simulink model "mainprueba3"  (R2016b)
settings: Solver=VariableStepAuto  StartTime=0.0  StopTime=10.0  MaxStep=0.2  RelTol=1e-2
undefined symbols (not defined in the file): checks, Earth, initialValues, LD, Newton, Raphson, WGS84
libraries: aerolibasang x5, aerolibutil x5, simulink x5, aerolibbdyn x3, aerolibatmos2 x1, aerolibobsolete x1, aerolibadyn x1, aerolibadynsys x1, aerolib6dof2 x1, aerolibtransform2 x1
(part 1 of 2)
settings Model: Creator=Uxío  LastModifiedBy=Uxío
settings DebuggingCC: ReadBeforeWriteMsg=DisableAll  WriteAfterWriteMsg=DisableAll  WriteAfterReadMsg=DisableAll  MultiTaskDSMMsg=none

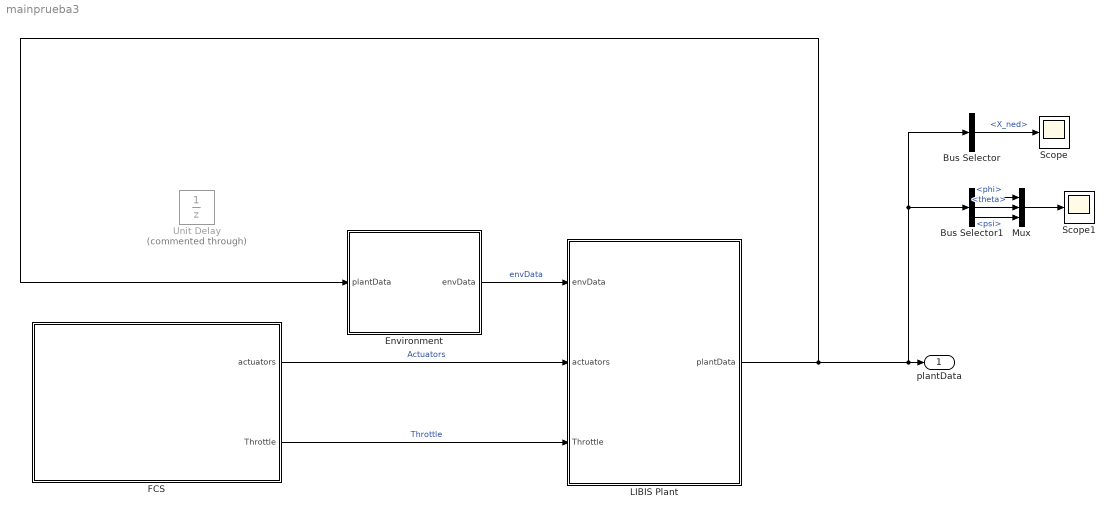
== system mainprueba3 ==
  Bus Selector : BusSelector  OutputSignals=X_ned
  Bus Selector1 : BusSelector  OutputSignals=Euler.phi,Euler.theta,Euler.psi
  Environment : Subsystem
      mask Display:
      | imageName='Wind.png';
      | currentPath=get_param(bdroot, 'FileName');
      | positions=strfind(currentPath,'\');
      | imagePath=strcat(currentPath(1:positions(end-1)),'graphics\',imageName);
      | image(imagePath);
  FCS : Subsystem
      mask Display:
      | imageName='FCS.png';
      | currentPath=get_param(bdroot, 'FileName');
      | positions=strfind(currentPath,'\');
      | imagePath=strcat(currentPath(1:positions(end-1)),'graphics\',imageName);
      | image(imagePath);
  LIBIS Plant : Subsystem
      mask Display:
      | imageName='LIBIS_Plant.jpg';
      | currentPath=get_param(bdroot, 'FileName');
      | positions=strfind(currentPath,'\');
      | imagePath=strcat(currentPath(1:positions(end-1)),'graphics\',imageName);
      | image(imagePath);
  Mux : Mux  Inputs=3
  Scope : Scope
  Scope1 : Scope
  Unit Delay : UnitDelay  Commented=through  SampleTime=-1
  plantData : Outport
  wires:
  LIBIS Plant/1(plantData) -> Environment/1(plantData), Bus Selector1/1, Bus Selector/1, plantData/1
  Environment/1(envData) -> LIBIS Plant/1(envData)  "envData"
  FCS/1(actuators) -> LIBIS Plant/2(actuators)  "Actuators"
  FCS/2(Throttle) -> LIBIS Plant/3(Throttle)  "Throttle"
  Bus Selector/1 -> Scope/1  "<X_ned>"
  Bus Selector1/1 -> Mux/1  "<phi>"
  Bus Selector1/2 -> Mux/2  "<theta>"
  Bus Selector1/3 -> Mux/3  "<psi>"
  Mux/1 -> Scope1/1

== system mainprueba3/Environment ==
  plantData : Inport
  Bus Selector : BusSelector  OutputSignals=X_ned,LLA.Altitude_m,V_ned,DCM_body_earth,LLA.Latitude_deg
  COESA Atmosphere Model : aerolibatmos2/COESA Atmosphere Model  units=Metric (MKS)  spec=1976 COESA-extended U.S. Standard Atmosphere  model=Profile  profile_var=High temperature  profile_percent=1%  profile_alt=5 km (16404 ft)  envelope_var=High temperature  envelope_percent=1%  action=Warning
  Gravity in Earth Axes : Gain  Gain=[0 0 LD.Inertia.mass]  SaturateOnIntegerOverflow=on  OutDataTypeStr=Inherit: Same as input  ParamDataTypeStr=Inherit: Same as input
  Math Function : Math  Operator=transpose  SaturateOnIntegerOverflow=on
  Terrain : Subsystem
  To Body Axes : Product  Multiplication=Matrix(*)  SaturateOnIntegerOverflow=on  InputSameDT=on  OutDataTypeStr=Inherit: Same as first input
  WGS84 Gravity Model : aerolibobsolete/WGS84 Gravity Model  model=WGS84 Taylor Series  units=Metric (MKS)  no_atmos=on  precessing=on  month=February  day=1  year=2000  no_centrifugal=on  action=Warning
  Wind Models : Subsystem
  envDataBus : BusCreator  Inputs='h_ground','windVelocity','windOmega','T','a','P','AirDensity','Fg'  OutDataTypeStr=Bus: envDataBus  NonVirtualBus=on
  envData : Outport  InitialOutput=0
  wires:
  [Altitude] -> COESA Atmosphere Model/1
  Bus Selector/4 -> Wind Models/3(DCM_be), To Body Axes/1  "<DCM_body_earth>"
  Bus Selector/5 -> WGS84 Gravity Model/2  "<Latitude_deg>"
  Bus Selector/3 -> Wind Models/1(Ve)  "<V_ned>"
  [Altitude] -> WGS84 Gravity Model/1
  envDataBus/1 -> envData/1  "envData"
  To Body Axes/1 -> envDataBus/8  "Fg"
  Wind Models/2(windOmega) -> envDataBus/3  "windOmega"
  Bus Selector/1 -> Terrain/1(Xe)  "<X_ned>"
  WGS84 Gravity Model/1 -> Gravity in Earth Axes/1
  COESA Atmosphere Model/3 -> envDataBus/6  "P"
  COESA Atmosphere Model/2 -> envDataBus/5  "a"
  Wind Models/1(windVelocity) -> envDataBus/2  "windVelocity"
  [Altitude] -> Wind Models/2(Altitude)
  COESA Atmosphere Model/1 -> envDataBus/4  "T"
  COESA Atmosphere Model/4 -> envDataBus/7  "AirDensity"
  plantData/1 -> Bus Selector/1
  Terrain/1(hground) -> envDataBus/1  "h_ground"
  Bus Selector/2 -> [Altitude]  "<Altitude_m>"
  Gravity in Earth Axes/1 -> Math Function/1
  Math Function/1 -> To Body Axes/2

== system mainprueba3/FCS ==
  Bus Creator : BusCreator  Inputs=4
  Bus Creator1 : BusCreator  Inputs=5
  Constant{,1..4} (5 alike) : Constant  Value=0
  Constant{5..8} (4 alike) : Constant
  actuators : Outport
  Throttle : Outport  Port=2
  wires:
  Bus Creator/1 -> actuators/1  "actuators"
  Constant/1 -> Bus Creator/1  "deltae"
  Constant1/1 -> Bus Creator/2  "deltar"
  Constant2/1 -> Bus Creator/3  "deltafr"
  Constant3/1 -> Bus Creator/4  "deltafl"
  Constant4/1 -> Bus Creator1/1  "Throttle1"
  Constant5/1 -> Bus Creator1/2  "Throttle2"
  Constant6/1 -> Bus Creator1/3  "Throttle3"
  Constant7/1 -> Bus Creator1/4  "Throttle4"
  Constant8/1 -> Bus Creator1/5  "Throttle5"
  Bus Creator1/1 -> Throttle/1

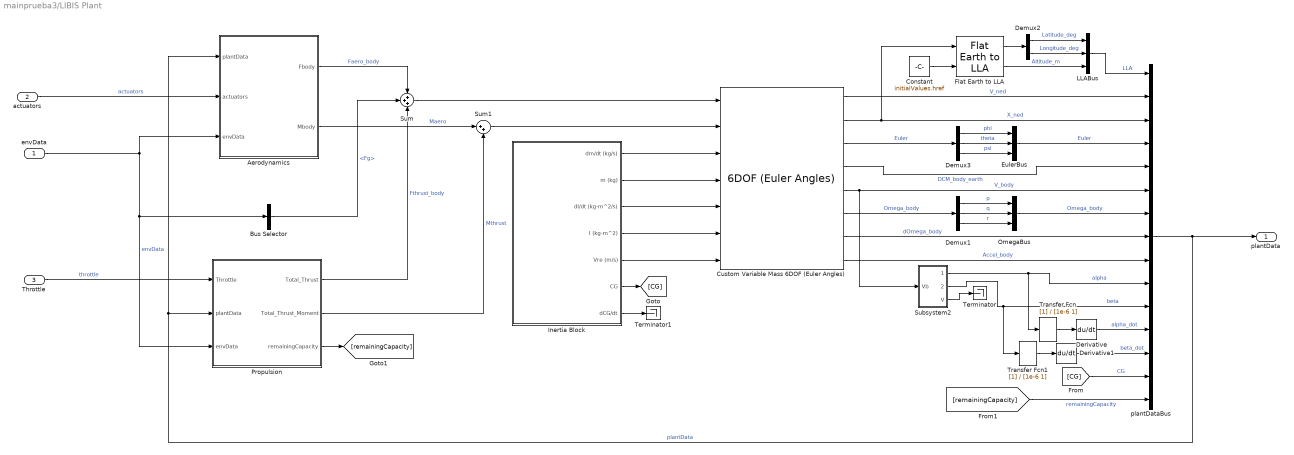
== system mainprueba3/LIBIS Plant ==
  envData : Inport
  actuators : Inport  Port=2
  Throttle : Inport  Port=3
  Aerodynamics : Subsystem
  Bus Selector : BusSelector  OutputSignals=Fg
  Constant : Constant  Value=initialValues.href
  Custom Variable Mass 6DOF (Euler Angles) : aerolib6dof2/6DOF (Euler Angles)  units=Metric (MKS)  mtype=Custom Variable  rep=Euler Angles  xme_0=[initialValues.Xe0 initialValues.Ye0 initialValues.Ze0]  Vm_0=[initialValues.u0 initialValues.v0 initialValues.w0]  eul_0=[initialValues.roll0 initialValues.pitch0 initialValues.yaw0]  pm_0=[initialValues.p0 initialValues.q0 initialValues.r0]  mass_0=1.0  mass_e=0.5  mass_f=2.0  inertia=eye(3)  inertia_e=eye(3)  inertia_f=2*eye(3)  k_quat=1.0  vre_flag=on
  Demux1 : Demux  Outputs=3
  Demux2 : Demux  Outputs=2
  Demux3 : Demux  Outputs=3
  Derivative : Derivative
  Derivative1 : Derivative
  EulerBus : BusCreator  Inputs='phi','theta','psi'  OutDataTypeStr=Bus: EulerBus  NonVirtualBus=on
  Flat Earth to LLA : aerolibtransform2/Flat Earth to LLA  units=Metric (MKS)  ptype=Earth (WGS84)  F=1/298.257223563  R=6378137  LL0=initialValues.LatLong0  psi=initialValues.heading0
  Inertia Block : Subsystem
      mask Display:
      | imageName='Moment_of_inertia.png';
      | currentPath=get_param(bdroot, 'FileName');
      | positions=strfind(currentPath,'\');
      | imagePath=strcat(currentPath(1:positions(end-1)),'graphics\',imageName);
      | image(imagePath);
  LLABus : BusCreator  Inputs='Latitude_deg','Longitude_deg','Altitude_m'  OutDataTypeStr=Bus: LLABus  NonVirtualBus=on
  OmegaBus : BusCreator  Inputs='p','q','r'  OutDataTypeStr=Bus: OmegaBus  NonVirtualBus=on
  Propulsion : Subsystem
  Subsystem2 : Subsystem
  Sum : Sum  Inputs=+++
  Sum1 : Sum  Inputs=|++
  Terminator : Terminator
  Terminator1 : Terminator
  Transfer Fcn : TransferFcn  Denominator=[1e-6 1]
  Transfer Fcn1 : TransferFcn  Denominator=[1e-6 1]
  plantDataBus : BusCreator  Inputs='LLA','V_ned','X_ned','Euler','DCM_body_earth','V_body','Omega_body','dOmega_body','Accel_body','alpha','beta','alpha_dot','beta_dot','CG','remainingCapacity'  OutDataTypeStr=Bus: plantDataBus  NonVirtualBus=on
  plantData : Outport
  wires:
  envData/1 -> Aerodynamics/3(envData), Propulsion/3(envData), Bus Selector/1  "envData"
  Inertia Block/4(I (kg-m^2)) -> Custom Variable Mass 6DOF (Euler Angles)/6
  Derivative1/1 -> plantDataBus/13  "beta_dot"
  plantDataBus/1 -> plantData/1, Propulsion/2(plantData), Aerodynamics/1(plantData)  "plantData"
  Flat Earth to LLA/2 -> LLABus/3  "Altitude_m"
  Custom Variable Mass 6DOF (Euler Angles)/2 -> plantDataBus/3, Flat Earth to LLA/1  "X_ned"
  Subsystem2/3(V) -> Terminator/1
  Custom Variable Mass 6DOF (Euler Angles)/3 -> Demux3/1  "Euler"
  EulerBus/1 -> plantDataBus/4  "Euler"
  Flat Earth to LLA/1 -> Demux2/1
  Demux2/1 -> LLABus/1  "Latitude_deg"
  Inertia Block/2(m (kg)) -> Custom Variable Mass 6DOF (Euler Angles)/4
  Inertia Block/5(Vre (m/s)) -> Custom Variable Mass 6DOF (Euler Angles)/7
  Custom Variable Mass 6DOF (Euler Angles)/5 -> Subsystem2/1(Vb), plantDataBus/6  "V_body"
  Inertia Block/7(dCG/dt) -> Terminator1/1
  [CG] -> plantDataBus/14  "CG"
  Custom Variable Mass 6DOF (Euler Angles)/4 -> plantDataBus/5  "DCM_body_earth"
  Inertia Block/3(dI/dt (kg-m^2/s)) -> Custom Variable Mass 6DOF (Euler Angles)/5
  LLABus/1 -> plantDataBus/1  "LLA"
  Custom Variable Mass 6DOF (Euler Angles)/8 -> plantDataBus/9  "Accel_body"
  Subsystem2/1(Alpha) -> Transfer Fcn/1, plantDataBus/10  "alpha"
  Demux3/1 -> EulerBus/1  "phi"
  Demux3/3 -> EulerBus/3  "psi"
  Inertia Block/6(CG) -> [CG]
  Inertia Block/1(dm/dt (kg/s)) -> Custom Variable Mass 6DOF (Euler Angles)/3
  Constant/1 -> Flat Earth to LLA/2
  Demux2/2 -> LLABus/2  "Longitude_deg"
  Custom Variable Mass 6DOF (Euler Angles)/7 -> plantDataBus/8  "dOmega_body"
  Subsystem2/2(Beta) -> Transfer Fcn1/1, plantDataBus/11  "beta"
  Demux3/2 -> EulerBus/2  "theta"
  Derivative/1 -> plantDataBus/12  "alpha_dot"
  Custom Variable Mass 6DOF (Euler Angles)/1 -> plantDataBus/2  "V_ned"
  OmegaBus/1 -> plantDataBus/7  "Omega_body"
  Custom Variable Mass 6DOF (Euler Angles)/6 -> Demux1/1  "Omega_body"
  Demux1/2 -> OmegaBus/2  "q"
  Demux1/1 -> OmegaBus/1  "p"
  Demux1/3 -> OmegaBus/3  "r"
  Aerodynamics/1(Fbody) -> Sum/1  "Faero_body"
  Sum1/1 -> Custom Variable Mass 6DOF (Euler Angles)/2
  Aerodynamics/2(Mbody) -> Sum1/1  "Maero"
  Propulsion/2(Total_Thrust_Moment) -> Sum1/2  "Mthrust"
  actuators/1 -> Aerodynamics/2(actuators)  "actuators"
  Throttle/1 -> Propulsion/1(Throttle)  "throttle"
  Propulsion/3(remainingCapacity) -> [remainingCapacity]
  [remainingCapacity] -> plantDataBus/15  "remainingCapacity"
  Propulsion/1(Total_Thrust) -> Sum/3  "Fthrust_body"
  Bus Selector/1 -> Sum/2  "<Fg>"
  Sum/1 -> Custom Variable Mass 6DOF (Euler Angles)/1
  Transfer Fcn1/1 -> Derivative1/1
  Transfer Fcn/1 -> Derivative/1

== system mainprueba3/Environment/Terrain ==
  note: This part of the system defines the interface for the terrain model that will be developed in detail later on.
  Xe : Inport
  Terminator : Terminator
  hground_value : Constant  Value=initialValues.href  OutDataTypeStr=double
  hground : Outport  Unit=m
  wires:
  Xe/1 -> Terminator/1
  hground_value/1 -> hground/1  "hground"

== system mainprueba3/Environment/Wind Models ==
  Ve : Inport
  Altitude : Inport  Port=2
  DCM_be : Inport  Port=3
  Constant : Constant  Value=[0,0,0]
  Constant1 : Constant  Value=[0,0,0]
  Dot Product : DotProduct  OutDataTypeStr=Inherit: Inherit via internal rule
  vt : Sqrt  SaturateOnIntegerOverflow=on
  windVelocity : Outport  Unit=m/s
  windOmega : Outport  Port=2  Unit=rad/second
  wires:
  DCM_be/1 -> [DCM]
  Altitude/1 -> [Altitude]
  vt/1 -> [Airspeed]  "Airspeed"
  Dot Product/1 -> vt/1
  Ve/1 -> Dot Product/2, Dot Product/1
  Constant/1 -> windVelocity/1
  Constant1/1 -> windOmega/1

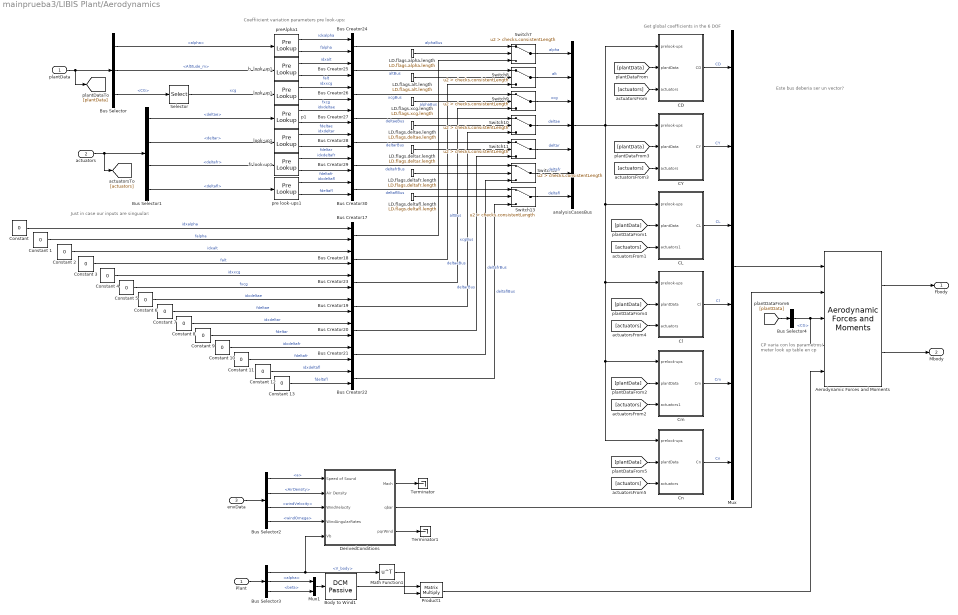
== system mainprueba3/LIBIS Plant/Aerodynamics ==
  note: Este bus deberia ser un vector?
  note: CP varia con los parametros! meter look up table en cp
  note: Just in case our inputs are singuular:
  note: Get global coefficients in the 6 DOF
  note: Coeffiicient variation parameters pre look-ups:
  plantData : Inport
  actuators : Inport  Port=2
  envData : Inport  Port=3
  " look-up1" : PreLookup  BreakpointsData=LD.xcg  BeginIndexSearchUsingPreviousIndexResult=on  IndexDataTypeStr=int32  FractionDataTypeStr=double
  "Aerodynamic Forces and Moments " : aerolibadyn/Aerodynamic Forces and Moments   inputAxes=Stability  outputForceAxes=Body  outputMomentAxes=Body  S=LD.sref  b=LD.blref  cbar=LD.cbar
  Body to Wind1 : aerolibadynsys/DCM Passive  SystemSampleTime=-1
  Bus Creator17 : BusCreator  Inputs='idxalpha','falpha'  OutDataTypeStr=Bus: alphaBus  NonVirtualBus=on
  Bus Creator18 : BusCreator  Inputs='idxalt','falt'  OutDataTypeStr=Bus: altBus  NonVirtualBus=on
  Bus Creator19 : BusCreator  Inputs='idxdeltae','fdeltae'  OutDataTypeStr=Bus: deltaeBus  NonVirtualBus=on
  Bus Creator20 : BusCreator  Inputs='idxdeltar','fdeltar'  OutDataTypeStr=Bus: deltarBus  NonVirtualBus=on
  Bus Creator21 : BusCreator  Inputs='idxdeltafr','fdeltafr'  OutDataTypeStr=Bus: deltafrBus  NonVirtualBus=on
  Bus Creator22 : BusCreator  Inputs='idxdeltafl','fdeltafl'  OutDataTypeStr=Bus: deltaflBus  NonVirtualBus=on
  Bus Creator23 : BusCreator  Inputs='idxxcg','fxcg'  OutDataTypeStr=Bus: xcgBus  NonVirtualBus=on
  Bus Creator24 : BusCreator  Inputs='idxalpha','falpha'  OutDataTypeStr=Bus: alphaBus  NonVirtualBus=on
  Bus Creator25 : BusCreator  Inputs='idxalt','falt'  OutDataTypeStr=Bus: altBus  NonVirtualBus=on
  Bus Creator26 : BusCreator  Inputs='idxxcg','fxcg'  OutDataTypeStr=Bus: xcgBus  NonVirtualBus=on
  Bus Creator27 : BusCreator  Inputs='idxdeltae','fdeltae'  OutDataTypeStr=Bus: deltaeBus  NonVirtualBus=on
  Bus Creator28 : BusCreator  Inputs='idxdeltar','fdeltar'  OutDataTypeStr=Bus: deltarBus  NonVirtualBus=on
  Bus Creator29 : BusCreator  Inputs='idxdeltafr','fdeltafr'  OutDataTypeStr=Bus: deltafrBus  NonVirtualBus=on
  Bus Creator30 : BusCreator  Inputs='idxdeltafl','fdeltafl'  OutDataTypeStr=Bus: deltaflBus  NonVirtualBus=on
  Bus Selector : BusSelector  OutputSignals=alpha,LLA.Altitude_m,CG
  Bus Selector1 : BusSelector  OutputSignals=deltae,deltar,deltafr,deltafl
  Bus Selector2 : BusSelector  OutputSignals=a,AirDensity,windVelocity,windOmega
  Bus Selector3 : BusSelector  OutputSignals=V_body,alpha,beta
  Bus Selector4 : BusSelector  OutputSignals=CG
  CD : Subsystem
  CL : Subsystem
  CY : Subsystem
  Cl : Subsystem
  Cm : Subsystem
  Cn : Subsystem
  Constant {,2,4,6,8,10,12} (7 alike) : Constant  Value=0  OutDataTypeStr=int32
  Constant {1,3,5,7,9,11,13} (7 alike) : Constant  Value=0
  DerivedConditions : Subsystem
  LD.flags.alpha.length : Constant  Value=LD.flags.alpha.length
  LD.flags.alt.length : Constant  Value=LD.flags.alt.length
  LD.flags.deltae.length : Constant  Value=LD.flags.deltae.length
  LD.flags.deltafl.length : Constant  Value=LD.flags.deltafl.length
  LD.flags.deltafr.length : Constant  Value=LD.flags.deltafr.length
  LD.flags.deltar.length : Constant  Value=LD.flags.deltar.length
  LD.flags.xcg.length : Constant  Value=LD.flags.xcg.length
  Math Function1 : Math  Operator=transpose  SaturateOnIntegerOverflow=on
  Mux : Mux  Inputs=6
  Mux1 : Mux  Inputs=2
  "Plant " : InportShadow
  Product1 : Product  Multiplication=Matrix(*)  RndMeth=Zero
  Selector : Selector  InputPortWidth=3  IndexOptions=Index vector (dialog)  Indices=[1 ]  OutputSizes=1
  Switch{7..13} (7 alike) : Switch  Criteria=u2 > Threshold  Threshold=checks.consistentLength
  Terminator : Terminator
  Terminator1 : Terminator
  analysisCasesBus : BusCreator  Inputs='alpha','alt','xcg','deltae','deltar','deltafr','deltafl'  OutDataTypeStr=Bus: analysisCasesBus  NonVirtualBus=on
  fr look-up1 : PreLookup  BreakpointsData=LD.deltafr  BeginIndexSearchUsingPreviousIndexResult=on  IndexDataTypeStr=int32  FractionDataTypeStr=double
  h  look-up1 : PreLookup  BreakpointsData=LD.alt  BeginIndexSearchUsingPreviousIndexResult=on  IndexDataTypeStr=int32  FractionDataTypeStr=double
  look-up1 : PreLookup  BreakpointsData=LD.deltar  BeginIndexSearchUsingPreviousIndexResult=on  IndexDataTypeStr=int32  FractionDataTypeStr=double
  p1 : PreLookup  BreakpointsData=LD.deltae  BeginIndexSearchUsingPreviousIndexResult=on  IndexDataTypeStr=int32  FractionDataTypeStr=double
  pre look-ups1 : PreLookup  BreakpointsData=LD.deltafl  BeginIndexSearchUsingPreviousIndexResult=on  IndexDataTypeStr=int32  FractionDataTypeStr=double
  preAlpha1 : PreLookup  BreakpointsData=LD.alpha  BeginIndexSearchUsingPreviousIndexResult=on  IndexDataTypeStr=int32  FractionDataTypeStr=double
  Fbody : Outport  Unit=N
  Mbody : Outport  Port=2  Unit=N*m
  wires:
  plantData/1 -> [plantData], Bus Selector/1
  Mux1/1 -> Body to Wind1/1
  preAlpha1/2 -> Bus Creator24/2  "falpha"
  preAlpha1/1 -> Bus Creator24/1  "idxalpha"
  h  look-up1/2 -> Bus Creator25/2  "falt"
  h  look-up1/1 -> Bus Creator25/1  "idxalt"
  " look-up1"/1 -> Bus Creator26/1  "idxxcg"
  " look-up1"/2 -> Bus Creator26/2  "fxcg"
  p1/2 -> Bus Creator27/2  "fdeltae"
  p1/1 -> Bus Creator27/1  "idxdeltae"
  look-up1/2 -> Bus Creator28/2  "fdeltar"
  look-up1/1 -> Bus Creator28/1  "idxdeltar"
  fr look-up1/2 -> Bus Creator29/2  "fdeltafr"
  fr look-up1/1 -> Bus Creator29/1  "idxdeltafr"
  pre look-ups1/1 -> Bus Creator30/1  "idxdeltafl"
  pre look-ups1/2 -> Bus Creator30/2  "fdeltafl"
  LD.flags.alpha.length/1 -> Switch7/2
  Bus Creator24/1 -> Switch7/1  "alphaBus"
  LD.flags.alt.length/1 -> Switch8/2
  Bus Creator25/1 -> Switch8/1  "altBus"
  LD.flags.xcg.length/1 -> Switch9/2
  Bus Creator26/1 -> Switch9/1  "xcgBus"
  LD.flags.deltae.length/1 -> Switch10/2
  Bus Creator27/1 -> Switch10/1  "deltaeBus"
  LD.flags.deltar.length/1 -> Switch11/2
  Bus Creator28/1 -> Switch11/1  "deltarBus"
  LD.flags.deltafr.length/1 -> Switch12/2
  Bus Creator29/1 -> Switch12/1  "deltafrBus"
  LD.flags.deltafl.length/1 -> Switch13/2
  Bus Creator30/1 -> Switch13/1  "deltaflBus"
  Bus Creator17/1 -> Switch7/3  "alphaBus"
  Bus Creator18/1 -> Switch8/3  "altBus"
  Bus Creator23/1 -> Switch9/3  "xcgBus"
  Bus Creator19/1 -> Switch10/3  "deltaeBus"
  Bus Creator20/1 -> Switch11/3  "deltarBus"
  Bus Creator21/1 -> Switch12/3  "deltafrBus"
  Bus Creator22/1 -> Switch13/3  "deltaflBus"
  Switch7/1 -> analysisCasesBus/1  "alpha"
  Switch8/1 -> analysisCasesBus/2  "alt"
  Switch9/1 -> analysisCasesBus/3  "xcg"
  Switch10/1 -> analysisCasesBus/4  "deltae"
  Switch11/1 -> analysisCasesBus/5  "deltar"
  Switch12/1 -> analysisCasesBus/6  "deltafr"
  Switch13/1 -> analysisCasesBus/7  "deltafl"
  Constant 1/1 -> Bus Creator17/2  "falpha"
  "Constant "/1 -> Bus Creator17/1  "idxalpha"
  Constant 3/1 -> Bus Creator18/2  "falt"
  Constant 2/1 -> Bus Creator18/1  "idxalt"
  Constant 4/1 -> Bus Creator23/1  "idxxcg"
  Constant 5/1 -> Bus Creator23/2  "fxcg"
  Constant 7/1 -> Bus Creator19/2  "fdeltae"
  Constant 6/1 -> Bus Creator19/1  "idxdeltae"
  Constant 9/1 -> Bus Creator20/2  "fdeltar"
  Constant 8/1 -> Bus Creator20/1  "idxdeltar"
  Constant 11/1 -> Bus Creator21/2  "fdeltafr"
  Constant 10/1 -> Bus Creator21/1  "idxdeltafr"
  Constant 12/1 -> Bus Creator22/1  "idxdeltafl"
  Constant 13/1 -> Bus Creator22/2  "fdeltafl"
  analysisCasesBus/1 -> CD/1(prelook-ups), CY/1(prelook-ups), CL/1(prelook-ups), Cl/1(prelook-ups), Cm/1(prelook-ups), Cn/1(prelook-ups)
  Bus Selector/1 -> preAlpha1/1  "<alpha>"
  Bus Selector/2 -> h  look-up1/1  "<Altitude_m>"
  Bus Selector/3 -> Selector/1  "<CG>"
  Selector/1 -> " look-up1"/1  "xcg"
  actuators/1 -> [actuators], Bus Selector1/1
  Bus Selector1/1 -> p1/1  "<deltae>"
  Bus Selector1/2 -> look-up1/1  "<deltar>"
  Bus Selector1/3 -> fr look-up1/1  "<deltafr>"
  Bus Selector1/4 -> pre look-ups1/1  "<deltafl>"
  [plantData] -> CD/2(plantData)
  [actuators] -> CD/3(actuators)
  [plantData] -> CL/2(plantData)
  [plantData] -> Cm/2(plantData)
  [plantData] -> CY/2(plantData)
  [actuators] -> CY/3(actuators)
  [plantData] -> Cl/2(plantData)
  [actuators] -> Cl/3(actuators)
  [plantData] -> Cn/2(plantData)
  [actuators] -> Cn/3(actuators)
  Cn/1(Cn) -> Mux/6  "Cn"
  Cl/1(Cl) -> Mux/4  "Cl"
  CL/1(CL) -> Mux/3  "CL"
  CY/1(CY) -> Mux/2  "CY"
  CD/1(CD) -> Mux/1  "CD"
  Cm/1(Cm) -> Mux/5  "Cm"
  Mux/1 -> "Aerodynamic Forces and Moments "/1
  "Aerodynamic Forces and Moments "/1 -> Fbody/1
  "Aerodynamic Forces and Moments "/2 -> Mbody/1
  envData/1 -> Bus Selector2/1
  Bus Selector2/1 -> DerivedConditions/1(Speed of Sound)  "<a>"
  Bus Selector2/2 -> DerivedConditions/2(Air Density)  "<AirDensity>"
  Bus Selector2/3 -> DerivedConditions/3(WindVelocity)  "<windVelocity>"
  Bus Selector2/4 -> DerivedConditions/4(WindAngularRates)  "<windOmega>"
  "Plant "/1 -> Bus Selector3/1
  Bus Selector3/1 -> DerivedConditions/5(Vb), Math Function1/1  "<V_body>"
  DerivedConditions/1(Mach) -> Terminator/1
  DerivedConditions/3("pqrWind ") -> Terminator1/1
  DerivedConditions/2(qbar) -> "Aerodynamic Forces and Moments "/2
  Product1/1 -> "Aerodynamic Forces and Moments "/5
  Bus Selector3/2 -> Mux1/1  "<alpha>"
  Bus Selector3/3 -> Mux1/2  "<beta>"
  [plantData] -> Bus Selector4/1
  Bus Selector4/1 -> "Aerodynamic Forces and Moments "/4, "Aerodynamic Forces and Moments "/3  "<CG>"
  [actuators] -> CL/3(actuators1)
  [actuators] -> Cm/3(actuators1)
  Body to Wind1/1 -> Product1/1
  Math Function1/1 -> Product1/2

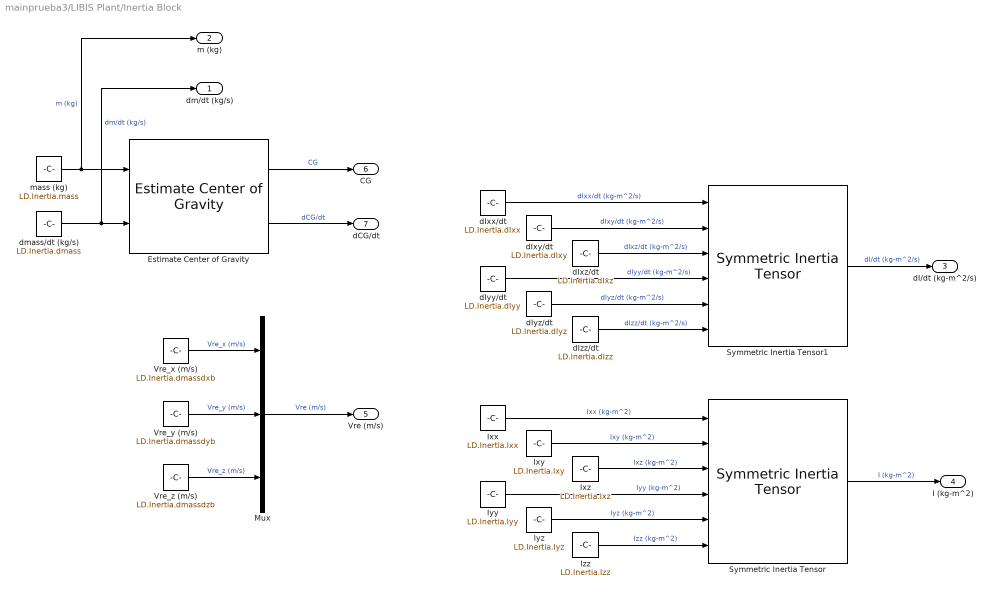
== system mainprueba3/LIBIS Plant/Inertia Block ==
  Estimate Center of Gravity : aerolibbdyn/Estimate Center of Gravity  fmass=LD.Inertia.fullMass  emass=LD.Inertia.emptyMass-1  fcg=LD.Inertia.fullCG  ecg=LD.Inertia.emptyCG
  Ixx : Constant  Value=LD.Inertia.Ixx
  Ixy : Constant  Value=LD.Inertia.Ixy
  Ixz : Constant  Value=LD.Inertia.Ixz
  Iyy : Constant  Value=LD.Inertia.Iyy
  Iyz : Constant  Value=LD.Inertia.Iyz
  Izz : Constant  Value=LD.Inertia.Izz
  Mux : Mux  Inputs=3
  Symmetric Inertia Tensor : aerolibbdyn/Symmetric Inertia Tensor
  Symmetric Inertia Tensor1 : aerolibbdyn/Symmetric Inertia Tensor
  Vre_x (m/s) : Constant  Value=LD.Inertia.dmassdxb
  Vre_y (m/s) : Constant  Value=LD.Inertia.dmassdyb
  Vre_z (m/s) : Constant  Value=LD.Inertia.dmassdzb
  dIxx/dt : Constant  Value=LD.Inertia.dIxx
  dIxy/dt : Constant  Value=LD.Inertia.dIxy
  dIxz/dt : Constant  Value=LD.Inertia.dIxz
  dIyy/dt : Constant  Value=LD.Inertia.dIyy
  dIyz/dt : Constant  Value=LD.Inertia.dIyz
  dIzz/dt : Constant  Value=LD.Inertia.dIzz
  dmass/dt (kg/s) : Constant  Value=LD.Inertia.dmass
  mass (kg) : Constant  Value=LD.Inertia.mass
  dm/dt (kg/s) : Outport  Unit=kg/s
  m (kg) : Outport  Port=2  Unit=kg
  dI/dt (kg-m^2/s) : Outport  Port=3  Unit=kg*meter^2/s
  I (kg-m^2) : Outport  Port=4  Unit=kg*meter*meter
  Vre (m/s) : Outport  Port=5  Unit=meter/s
  CG : Outport  Port=6
  dCG/dt : Outport  Port=7
  wires:
  Symmetric Inertia Tensor/1 -> I (kg-m^2)/1  "I (kg-m^2)"
  Symmetric Inertia Tensor1/1 -> dI/dt (kg-m^2/s)/1  "dI/dt (kg-m^2/s)"
  dIxx/dt/1 -> Symmetric Inertia Tensor1/1  "dIxx/dt (kg-m^2/s)"
  dIxz/dt/1 -> Symmetric Inertia Tensor1/3  "dIxz/dt (kg-m^2/s)"
  dIxy/dt/1 -> Symmetric Inertia Tensor1/2  "dIxy/dt (kg-m^2/s)"
  dIyy/dt/1 -> Symmetric Inertia Tensor1/4  "dIyy/dt (kg-m^2/s)"
  dIzz/dt/1 -> Symmetric Inertia Tensor1/6  "dIzz/dt (kg-m^2/s)"
  dIyz/dt/1 -> Symmetric Inertia Tensor1/5  "dIyz/dt (kg-m^2/s)"
  Ixx/1 -> Symmetric Inertia Tensor/1  "Ixx (kg-m^2)"
  Ixz/1 -> Symmetric Inertia Tensor/3  "Ixz (kg-m^2)"
  Ixy/1 -> Symmetric Inertia Tensor/2  "Ixy (kg-m^2)"
  Iyy/1 -> Symmetric Inertia Tensor/4  "Iyy (kg-m^2)"
  Izz/1 -> Symmetric Inertia Tensor/6  "Izz (kg-m^2)"
  Iyz/1 -> Symmetric Inertia Tensor/5  "Iyz (kg-m^2)"
  mass (kg)/1 -> m (kg)/1, Estimate Center of Gravity/1  "m (kg)"
  dmass/dt (kg/s)/1 -> Estimate Center of Gravity/2, dm/dt (kg/s)/1  "dm/dt (kg/s)"
  Vre_x (m/s)/1 -> Mux/1  "Vre_x (m/s)"
  Vre_z (m/s)/1 -> Mux/3  "Vre_z (m/s)"
  Vre_y (m/s)/1 -> Mux/2  "Vre_y (m/s)"
  Mux/1 -> Vre (m/s)/1  "Vre (m/s)"
  Estimate Center of Gravity/1 -> CG/1  "CG"
  Estimate Center of Gravity/2 -> dCG/dt/1  "dCG/dt"

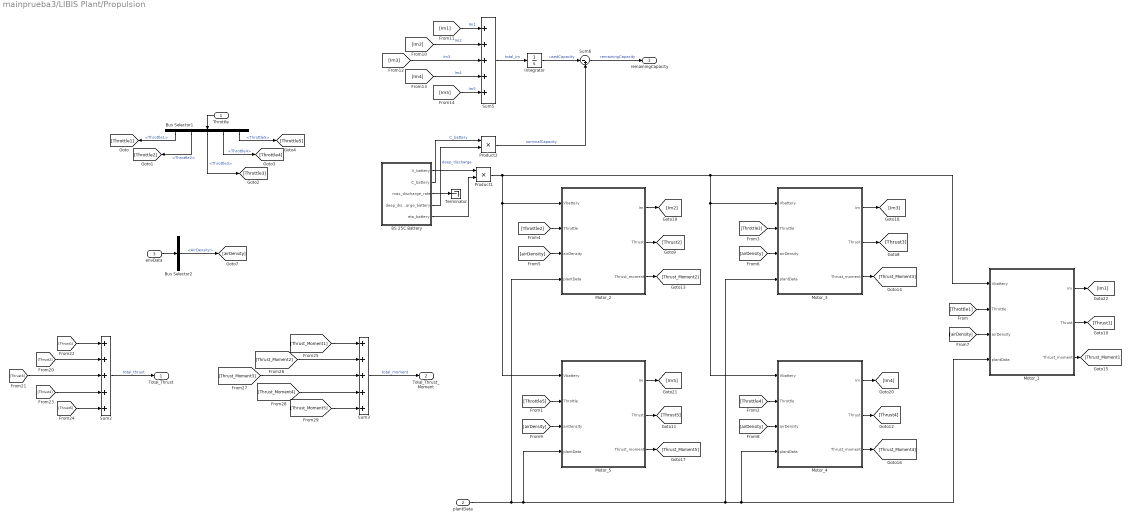
== system mainprueba3/LIBIS Plant/Propulsion ==
  Throttle : Inport
  plantData : Inport  Port=2
  envData : Inport  Port=3
  8S 25C Battery : Subsystem
  Bus Selector1 : BusSelector  OutputSignals=Throttle1,Throttle2,Throttle3,Throttle4,Throttle5
  Bus Selector2 : BusSelector  OutputSignals=AirDensity
  Integrator : Integrator
  Motor_1 : Subsystem
      mask Display:
      | imageName='LIBIS_Motor1.png';
      | currentPath=get_param(bdroot, 'FileName');
      | positions=strfind(currentPath,'\');
      | imagePath=strcat(currentPath(1:positions(end-1)),'graphics\',imageName);
      | image(imagePath);
  Motor_2 : Subsystem
      mask Display:
      | imageName='LIBIS_Motor2.png';
      | currentPath=get_param(bdroot, 'FileName');
      | positions=strfind(currentPath,'\');
      | imagePath=strcat(currentPath(1:positions(end-1)),'graphics\',imageName);
      | image(imagePath);
  Motor_3 : Subsystem
      mask Display:
      | imageName='LIBIS_Motor3.png';
      | currentPath=get_param(bdroot, 'FileName');
      | positions=strfind(currentPath,'\');
      | imagePath=strcat(currentPath(1:positions(end-1)),'graphics\',imageName);
      | image(imagePath);
  Motor_4 : Subsystem
      mask Display:
      | imageName='LIBIS_Motor4.png';
      | currentPath=get_param(bdroot, 'FileName');
      | positions=strfind(currentPath,'\');
      | imagePath=strcat(currentPath(1:positions(end-1)),'graphics\',imageName);
      | image(imagePath);
  Motor_5 : Subsystem
      mask Display:
      | imageName='LIBIS_Motor5.png';
      | currentPath=get_param(bdroot, 'FileName');
      | positions=strfind(currentPath,'\');
      | imagePath=strcat(currentPath(1:positions(end-1)),'graphics\',imageName);
      | image(imagePath);
  Product1 : Product
  Product2 : Product
  Sum2 : Sum  Inputs=+++++
  Sum3 : Sum  Inputs=+++++
  Sum5 : Sum  Inputs=+++++
  Sum6 : Sum  Inputs=|-+
  Terminator : Terminator
  Total_Thrust : Outport
  Total_Thrust_Moment : Outport  Port=2
  remainingCapacity : Outport  Port=3
  wires:
  Throttle/1 -> Bus Selector1/1
  Bus Selector1/1 -> [Throttle1]  "<Throttle1>"
  Bus Selector1/2 -> [Throttle2]  "<Throttle2>"
  Bus Selector1/3 -> [Throttle3]  "<Throttle3>"
  Bus Selector1/4 -> [Throttle4]  "<Throttle4>"
  Bus Selector1/5 -> [Throttle5]  "<Throttle5>"
  8S 25C Battery/1(V_battery) -> Product1/1
  8S 25C Battery/5(eta_battery) -> Product1/2
  8S 25C Battery/2(C_battery) -> Product2/1  "C_battery"
  8S 25C Battery/3(max_discharge_rate) -> Terminator/1
  8S 25C Battery/4(deep_discharge_battery) -> Product2/2  "deep_discharge"
  envData/1 -> Bus Selector2/1
  Bus Selector2/1 -> [airDensity]  "<AirDensity>"
  [Throttle1] -> Motor_1/2(Throttle)
  [Throttle2] -> Motor_2/2(Throttle)
  Product1/1 -> Motor_1/1(Vbattery), Motor_3/1(Vbattery), Motor_4/1(Vbattery), Motor_2/1(Vbattery), Motor_5/1(Vbattery)
  [Throttle5] -> Motor_5/2(Throttle)
  [Throttle4] -> Motor_4/2(Throttle)
  [Throttle3] -> Motor_3/2(Throttle)
  [airDensity] -> Motor_5/3(airDensity)
  [airDensity] -> Motor_4/3(airDensity)
  [airDensity] -> Motor_1/3(airDensity)
  [airDensity] -> Motor_3/3(airDensity)
  [airDensity] -> Motor_2/3(airDensity)
  Motor_3/2(Thrust) -> [Thrust3]
  Motor_2/2(Thrust) -> [Thrust2]
  Motor_1/2(Thrust) -> [Thrust1]
  Motor_4/2(Thrust) -> [Thrust4]
  Motor_5/2(Thrust) -> [Thrust5]
  [Thrust1] -> Sum2/1
  [Thrust2] -> Sum2/2
  [Thrust3] -> Sum2/3
  [Thrust4] -> Sum2/4
  [Thrust5] -> Sum2/5
  Sum2/1 -> Total_Thrust/1  "total_thrust"
  Sum3/1 -> Total_Thrust_Moment/1  "total_moment"
  Motor_2/3(Thrust_moment) -> [Thrust_Moment2]
  Motor_1/3(Thrust_moment) -> [Thrust_Moment1]
  Motor_3/3(Thrust_moment) -> [Thrust_Moment3]
  [Thrust_Moment1] -> Sum3/1
  [Thrust_Moment2] -> Sum3/2
  [Thrust_Moment3] -> Sum3/3
  Motor_4/3(Thrust_moment) -> [Thrust_Moment4]
  [Thrust_Moment4] -> Sum3/4
  Motor_5/3(Thrust_moment) -> [Thrust_Moment5]
  [Thrust_Moment5] -> Sum3/5
  Product2/1 -> Sum6/2  "nominalCapacity"
  Motor_3/1(Im) -> [Im3]
  Motor_1/1(Im) -> [Im1]
  Motor_5/1(Im) -> [Im5]
  Motor_4/1(Im) -> [Im4]
  Motor_2/1(Im) -> [Im2]
  plantData/1 -> Motor_3/4(plantData), Motor_4/4(plantData), Motor_1/4(plantData), Motor_5/4(plantData), Motor_2/4(plantData)
  [Im3] -> Sum5/3  "Im3"
  [Im2] -> Sum5/2  "Im2"
  [Im1] -> Sum5/1  "Im1"
  [Im4] -> Sum5/4  "Im4"
  [Im5] -> Sum5/5  "Im5"
  Sum5/1 -> Integrator/1  "total_Im"
  Integrator/1 -> Sum6/1  "usedCapacity"
  Sum6/1 -> remainingCapacity/1  "remainingCapacity"

== system mainprueba3/LIBIS Plant/Subsystem2 ==
  Vb : Inport
  Airspeed : Sqrt  AlgorithmType=Newton-Raphson  SaturateOnIntegerOverflow=on
  Allow All : UnitConfiguration  UnitSystemsStr=English,SI,SI (extended)  AllowAllUnitSystems=off
  Constant : Constant  Value=0
  Incidence : Trigonometry  Operator=atan2
  Product : Product  Inputs=*/  SaturateOnIntegerOverflow=on  OutDataTypeStr=Inherit: Same as first input
  Sideslip : Trigonometry  Operator=asin
  Subsystem : aerolibasang/Incidence, Sideslip, & Airspeed/Subsystem
  Subsystem1 : aerolibasang/Incidence, Sideslip, & Airspeed/Subsystem1
  Switch : Switch  Criteria=u2 > Threshold
  dot : aerolibasang/Incidence, Sideslip, & Airspeed/dot
  Alpha : Outport  Unit=rad  InitialOutput=0
  Beta : Outport  Port=2  Unit=rad  InitialOutput=0
  V : Outport  Port=3  InitialOutput=0
  wires:
  Subsystem/2 -> Incidence/2
  Subsystem/1 -> Incidence/1
  Incidence/1 -> Alpha/1
  Subsystem1/1 -> Product/1
  dot/1 -> Airspeed/1
  Airspeed/1 -> V/1, Switch/2, Product/2
  Vb/1 -> Subsystem/1, Subsystem1/1, dot/1
  Sideslip/1 -> Beta/1
  Product/1 -> Switch/1
  Switch/1 -> Sideslip/1
  Constant/1 -> Switch/3

== system mainprueba3/LIBIS Plant/Aerodynamics/CD ==
  prelook-ups : Inport
  plantData : Inport  Port=2
  actuators : Inport  Port=3
  Add : Sum  Inputs=+++++++
  Bus Selector : BusSelector  OutputSignals=alpha,alpha_dot,Omega_body.q
  Bus Selector1 : BusSelector  OutputSignals=alpha,alt,xcg,deltae,deltar,deltafr,deltafl
  Bus Selector2 : BusSelector  OutputSignals=deltae,deltafr,deltafl
  CD0 : Interpolation_n-D  NumberOfTableDimensions=7  Table=LD.Stability.CD0  RequireIndexFractionAsBus=on  InternalRulePriority=Speed
      settings: InputPortMap=u0,u1,u2,u3,u4,u5,u6
  CDalpha : Interpolation_n-D  NumberOfTableDimensions=7  Table=LD.Stability.CDalpha  RequireIndexFractionAsBus=on  InternalRulePriority=Speed
      settings: InputPortMap=u0,u1,u2,u3,u4,u5,u6
  CDalpha_dot : Interpolation_n-D  NumberOfTableDimensions=7  Table=LD.Stability.CDalpha_dot  RequireIndexFractionAsBus=on  InternalRulePriority=Speed
      settings: InputPortMap=u0,u1,u2,u3,u4,u5,u6
  CDdeltae : Interpolation_n-D  NumberOfTableDimensions=7  Table=LD.Stability.CDdeltae  RequireIndexFractionAsBus=on  InternalRulePriority=Speed
      settings: InputPortMap=u0,u1,u2,u3,u4,u5,u6
  CDdeltafl : Interpolation_n-D  NumberOfTableDimensions=7  Table=LD.Stability.CDdeltafl  RequireIndexFractionAsBus=on  InternalRulePriority=Speed
      settings: InputPortMap=u0,u1,u2,u3,u4,u5,u6
  CDdeltafr : Interpolation_n-D  NumberOfTableDimensions=7  Table=LD.Stability.CDdeltafr  RequireIndexFractionAsBus=on  InternalRulePriority=Speed
      settings: InputPortMap=u0,u1,u2,u3,u4,u5,u6
  CDq : Interpolation_n-D  NumberOfTableDimensions=7  Table=LD.Stability.CDq  RequireIndexFractionAsBus=on  InternalRulePriority=Speed
      settings: InputPortMap=u0,u1,u2,u3,u4,u5,u6
  Product{,1..5} (6 alike) : Product
  CD : Outport
  wires:
  prelook-ups/1 -> Bus Selector1/1
  CD0/1 -> Add/1
  Add/1 -> CD/1
  plantData/1 -> Bus Selector/1
  actuators/1 -> Bus Selector2/1
  CDalpha/1 -> Product/1
  Product/1 -> Add/2
  Bus Selector/1 -> Product/2  "<alpha>"
  Bus Selector2/1 -> Product3/2  "<deltae>"
  CDdeltae/1 -> Product3/1
  Product3/1 -> Add/5
  Product2/1 -> Add/4
  Product1/1 -> Add/3
  CDalpha_dot/1 -> Product1/1
  CDq/1 -> Product2/1
  Bus Selector/3 -> Product2/2  "<q>"
  Bus Selector/2 -> Product1/2  "<alpha_dot>"
  Bus Selector1/7 -> CD0/7, CDdeltafl/7, CDdeltafr/7, CDdeltae/7, CDq/7, CDalpha_dot/7, CDalpha/7  "<deltafl>"
  Bus Selector1/6 -> CD0/6, CDdeltafl/6, CDdeltafr/6, CDdeltae/6, CDq/6, CDalpha_dot/6, CDalpha/6  "<deltafr>"
  Bus Selector1/5 -> CD0/5, CDdeltafl/5, CDdeltafr/5, CDdeltae/5, CDq/5, CDalpha_dot/5, CDalpha/5  "<deltar>"
  Bus Selector1/4 -> CD0/4, CDdeltafl/4, CDdeltafr/4, CDdeltae/4, CDq/4, CDalpha_dot/4, CDalpha/4  "<deltae>"
  Bus Selector1/2 -> CD0/2, CDdeltafl/2, CDdeltafr/2, CDdeltae/2, CDq/2, CDalpha_dot/2, CDalpha/2  "<alt>"
  Bus Selector1/3 -> CD0/3, CDdeltafl/3, CDdeltafr/3, CDdeltae/3, CDq/3, CDalpha_dot/3, CDalpha/3  "<xcg>"
  Bus Selector1/1 -> CD0/1, CDdeltafl/1, CDdeltafr/1, CDdeltae/1, CDq/1, CDalpha_dot/1, CDalpha/1  "<alpha>"
  Bus Selector2/3 -> Product5/2  "<deltafl>"
  CDdeltafl/1 -> Product5/1
  Product5/1 -> Add/7
  Product4/1 -> Add/6
  CDdeltafr/1 -> Product4/1
  Bus Selector2/2 -> Product4/2  "<deltafr>"

== system mainprueba3/LIBIS Plant/Aerodynamics/CL ==
  prelook-ups : Inport
  plantData : Inport  Port=2
  actuators1 : Inport  Port=3
  Add : Sum  Inputs=+++++++
  Bus Selector : BusSelector  OutputSignals=alpha,alpha_dot,Omega_body.q
  Bus Selector1 : BusSelector  OutputSignals=alpha,alt,xcg,deltae,deltar,deltafr,deltafl
  Bus Selector3 : BusSelector  OutputSignals=deltae,deltafr,deltafl
  CL0 : Interpolation_n-D  NumberOfTableDimensions=7  Table=LD.Stability.CL0  RequireIndexFractionAsBus=on  InternalRulePriority=Speed
      settings: InputPortMap=u0,u1,u2,u3,u4,u5,u6
  CLalpha : Interpolation_n-D  NumberOfTableDimensions=7  Table=LD.Stability.CLalpha  RequireIndexFractionAsBus=on  InternalRulePriority=Speed
      settings: InputPortMap=u0,u1,u2,u3,u4,u5,u6
  CLalpha_dot : Interpolation_n-D  NumberOfTableDimensions=7  Table=LD.Stability.CLalpha_dot  RequireIndexFractionAsBus=on  InternalRulePriority=Speed
      settings: InputPortMap=u0,u1,u2,u3,u4,u5,u6
  CLdeltae : Interpolation_n-D  NumberOfTableDimensions=7  Table=LD.Stability.CLdeltae  RequireIndexFractionAsBus=on  InternalRulePriority=Speed
      settings: InputPortMap=u0,u1,u2,u3,u4,u5,u6
  CLdeltafl : Interpolation_n-D  NumberOfTableDimensions=7  Table=LD.Stability.CLdeltafl  RequireIndexFractionAsBus=on  InternalRulePriority=Speed
      settings: InputPortMap=u0,u1,u2,u3,u4,u5,u6
  CLdeltafr : Interpolation_n-D  NumberOfTableDimensions=7  Table=LD.Stability.CLdeltafr  RequireIndexFractionAsBus=on  InternalRulePriority=Speed
      settings: InputPortMap=u0,u1,u2,u3,u4,u5,u6
  CLq : Interpolation_n-D  NumberOfTableDimensions=7  Table=LD.Stability.CLq  RequireIndexFractionAsBus=on  InternalRulePriority=Speed
      settings: InputPortMap=u0,u1,u2,u3,u4,u5,u6
  Product{,1..5} (6 alike) : Product
  CL : Outport
  wires:
  prelook-ups/1 -> Bus Selector1/1
  CL0/1 -> Add/1
  Add/1 -> CL/1
  plantData/1 -> Bus Selector/1
  CLalpha/1 -> Product/1
  CLalpha_dot/1 -> Product1/1
  CLq/1 -> Product2/1
  CLdeltae/1 -> Product3/1
  Product/1 -> Add/2
  Product1/1 -> Add/3
  Product2/1 -> Add/4
  Product3/1 -> Add/5
  Bus Selector/1 -> Product/2  "<alpha>"
  Bus Selector/2 -> Product1/2  "<alpha_dot>"
  Bus Selector/3 -> Product2/2  "<q>"
  actuators1/1 -> Bus Selector3/1
  Bus Selector3/3 -> Product5/2  "<deltafl>"
  CLdeltafl/1 -> Product5/1
  Product5/1 -> Add/7
  Product4/1 -> Add/6
  CLdeltafr/1 -> Product4/1
  Bus Selector3/2 -> Product4/2  "<deltafr>"
  Bus Selector3/1 -> Product3/2  "<deltae>"
  Bus Selector1/7 -> CL0/7, CLalpha/7, CLalpha_dot/7, CLdeltafl/7, CLdeltafr/7, CLdeltae/7, CLq/7  "<deltafl>"
  Bus Selector1/6 -> CL0/6, CLalpha/6, CLalpha_dot/6, CLdeltafl/6, CLdeltafr/6, CLdeltae/6, CLq/6  "<deltafr>"
  Bus Selector1/5 -> CL0/5, CLalpha/5, CLalpha_dot/5, CLdeltafl/5, CLdeltafr/5, CLdeltae/5, CLq/5  "<deltar>"
  Bus Selector1/4 -> CL0/4, CLalpha/4, CLalpha_dot/4, CLq/4, CLdeltafl/4, CLdeltafr/4, CLdeltae/4  "<deltae>"
  Bus Selector1/2 -> CL0/2, CLalpha/2, CLalpha_dot/2, CLq/2, CLdeltafl/2, CLdeltafr/2, CLdeltae/2  "<alt>"
  Bus Selector1/3 -> CL0/3, CLalpha/3, CLalpha_dot/3, CLq/3, CLdeltafl/3, CLdeltafr/3, CLdeltae/3  "<xcg>"
  Bus Selector1/1 -> CL0/1, CLalpha/1, CLalpha_dot/1, CLq/1, CLdeltafl/1, CLdeltafr/1, CLdeltae/1  "<alpha>"

== system mainprueba3/LIBIS Plant/Aerodynamics/CY ==
  prelook-ups : Inport
  plantData : Inport  Port=2
  actuators : Inport  Port=3
  Add : Sum  Inputs=++++++
  Bus Selector : BusSelector  OutputSignals=beta,Omega_body.p,Omega_body.r
  Bus Selector1 : BusSelector  OutputSignals=alpha,alt,xcg,deltae,deltar,deltafr,deltafl
  Bus Selector2 : BusSelector  OutputSignals=deltar,deltafr,deltafl
  CYbeta : Interpolation_n-D  NumberOfTableDimensions=7  Table=LD.Stability.CYbeta  RequireIndexFractionAsBus=on  InternalRulePriority=Speed
      settings: InputPortMap=u0,u1,u2,u3,u4,u5,u6
  "CYdeltafl " : Interpolation_n-D  NumberOfTableDimensions=7  Table=LD.Stability.CYdeltafl  RequireIndexFractionAsBus=on  InternalRulePriority=Speed
      settings: InputPortMap=u0,u1,u2,u3,u4,u5,u6
  "CYdeltafr " : Interpolation_n-D  NumberOfTableDimensions=7  Table=LD.Stability.CYdeltafr  RequireIndexFractionAsBus=on  InternalRulePriority=Speed
      settings: InputPortMap=u0,u1,u2,u3,u4,u5,u6
  CYdeltar : Interpolation_n-D  NumberOfTableDimensions=7  Table=LD.Stability.CYdeltar  RequireIndexFractionAsBus=on  InternalRulePriority=Speed
      settings: InputPortMap=u0,u1,u2,u3,u4,u5,u6
  CYp : Interpolation_n-D  NumberOfTableDimensions=7  Table=LD.Stability.CYp  RequireIndexFractionAsBus=on  InternalRulePriority=Speed
      settings: InputPortMap=u0,u1,u2,u3,u4,u5,u6
  CYr : Interpolation_n-D  NumberOfTableDimensions=7  Table=LD.Stability.CYr  RequireIndexFractionAsBus=on  InternalRulePriority=Speed
      settings: InputPortMap=u0,u1,u2,u3,u4,u5,u6
  Product{,1..5} (6 alike) : Product
  CY : Outport
  wires:
  Bus Selector1/7 -> "CYdeltafl "/7, "CYdeltafr "/7, CYdeltar/7, CYr/7, CYp/7, CYbeta/7  "<deltafl>"
  Bus Selector1/6 -> "CYdeltafl "/6, "CYdeltafr "/6, CYdeltar/6, CYr/6, CYp/6, CYbeta/6  "<deltafr>"
  Bus Selector1/5 -> "CYdeltafl "/5, "CYdeltafr "/5, CYdeltar/5, CYr/5, CYp/5, CYbeta/5  "<deltar>"
  prelook-ups/1 -> Bus Selector1/1
  Bus Selector1/4 -> "CYdeltafl "/4, "CYdeltafr "/4, CYdeltar/4, CYr/4, CYp/4, CYbeta/4  "<deltae>"
  Bus Selector1/2 -> "CYdeltafl "/2, "CYdeltafr "/2, CYdeltar/2, CYr/2, CYp/2, CYbeta/2  "<alt>"
  Bus Selector1/3 -> "CYdeltafl "/3, "CYdeltafr "/3, CYdeltar/3, CYr/3, CYp/3, CYbeta/3  "<xcg>"
  Bus Selector1/1 -> "CYdeltafl "/1, "CYdeltafr "/1, CYdeltar/1, CYr/1, CYp/1, CYbeta/1  "<alpha>"
  Add/1 -> CY/1
  plantData/1 -> Bus Selector/1
  actuators/1 -> Bus Selector2/1
  CYbeta/1 -> Product/1
  Product/1 -> Add/1
  Bus Selector/1 -> Product/2  "<beta>"
  Bus Selector2/1 -> Product3/2  "<deltar>"
  CYdeltar/1 -> Product3/1
  Product3/1 -> Add/4
  Product2/1 -> Add/3
  Product1/1 -> Add/2
  CYp/1 -> Product1/1
  CYr/1 -> Product2/1
  Bus Selector/3 -> Product2/2  "<r>"
  Bus Selector/2 -> Product1/2  "<p>"
  "CYdeltafl "/1 -> Product5/1
  Product5/1 -> Add/6
  Product4/1 -> Add/5
  "CYdeltafr "/1 -> Product4/1
  Bus Selector2/2 -> Product4/2  "<deltafr>"
  Bus Selector2/3 -> Product5/2  "<deltafl>"

== system mainprueba3/LIBIS Plant/Aerodynamics/Cl ==
  prelook-ups : Inport
  plantData : Inport  Port=2
  actuators : Inport  Port=3
  Add : Sum  Inputs=++++++
  Bus Selector : BusSelector  OutputSignals=beta,Omega_body.p,Omega_body.r
  Bus Selector1 : BusSelector  OutputSignals=alpha,alt,xcg,deltae,deltar,deltafr,deltafl
  Bus Selector2 : BusSelector  OutputSignals=deltar,deltafr,deltafl
  Clbeta : Interpolation_n-D  NumberOfTableDimensions=7  Table=LD.Stability.Clbeta  RequireIndexFractionAsBus=on  InternalRulePriority=Speed
      settings: InputPortMap=u0,u1,u2,u3,u4,u5,u6
  "Cldeltafl " : Interpolation_n-D  NumberOfTableDimensions=7  Table=LD.Stability.Cldeltafl  RequireIndexFractionAsBus=on  InternalRulePriority=Speed
      settings: InputPortMap=u0,u1,u2,u3,u4,u5,u6
  "Cldeltafr " : Interpolation_n-D  NumberOfTableDimensions=7  Table=LD.Stability.Cldeltafr  RequireIndexFractionAsBus=on  InternalRulePriority=Speed
      settings: InputPortMap=u0,u1,u2,u3,u4,u5,u6
  Cldeltar : Interpolation_n-D  NumberOfTableDimensions=7  Table=LD.Stability.Cldeltar  RequireIndexFractionAsBus=on  InternalRulePriority=Speed
      settings: InputPortMap=u0,u1,u2,u3,u4,u5,u6
  Clp : Interpolation_n-D  NumberOfTableDimensions=7  Table=LD.Stability.Clp  RequireIndexFractionAsBus=on  InternalRulePriority=Speed
      settings: InputPortMap=u0,u1,u2,u3,u4,u5,u6
  Clr : Interpolation_n-D  NumberOfTableDimensions=7  Table=LD.Stability.Clr  RequireIndexFractionAsBus=on  InternalRulePriority=Speed
      settings: InputPortMap=u0,u1,u2,u3,u4,u5,u6
  Product{,1..5} (6 alike) : Product
  Cl : Outport
  wires:
  Bus Selector1/7 -> Clbeta/7, Clp/7, Clr/7, Cldeltar/7, "Cldeltafr "/7, "Cldeltafl "/7  "<deltafl>"
  Bus Selector1/6 -> Clbeta/6, Clp/6, Clr/6, Cldeltar/6, "Cldeltafr "/6, "Cldeltafl "/6  "<deltafr>"
  Bus Selector1/5 -> Clbeta/5, Clp/5, Clr/5, Cldeltar/5, "Cldeltafr "/5, "Cldeltafl "/5  "<deltar>"
  prelook-ups/1 -> Bus Selector1/1
  Bus Selector1/4 -> Clbeta/4, Clp/4, Clr/4, Cldeltar/4, "Cldeltafr "/4, "Cldeltafl "/4  "<deltae>"
  Bus Selector1/2 -> Clbeta/2, Clp/2, Clr/2, Cldeltar/2, "Cldeltafr "/2, "Cldeltafl "/2  "<alt>"
  Bus Selector1/3 -> Clbeta/3, Clp/3, Clr/3, Cldeltar/3, "Cldeltafr "/3, "Cldeltafl "/3  "<xcg>"
  Bus Selector1/1 -> Clbeta/1, Clp/1, Clr/1, Cldeltar/1, "Cldeltafr "/1, "Cldeltafl "/1  "<alpha>"
  Add/1 -> Cl/1
  Clbeta/1 -> Product/1
  Product/1 -> Add/1
  Bus Selector/1 -> Product/2  "<beta>"
  Bus Selector2/1 -> Product3/2  "<deltar>"
  Cldeltar/1 -> Product3/1
  Product3/1 -> Add/4
  Product2/1 -> Add/3
  Product1/1 -> Add/2
  Clp/1 -> Product1/1
  Clr/1 -> Product2/1
  Bus Selector/3 -> Product2/2  "<r>"
  Bus Selector/2 -> Product1/2  "<p>"
  "Cldeltafl "/1 -> Product5/1
  Product5/1 -> Add/6
  Product4/1 -> Add/5
  "Cldeltafr "/1 -> Product4/1
  Bus Selector2/2 -> Product4/2  "<deltafr>"
  Bus Selector2/3 -> Product5/2  "<deltafl>"
  plantData/1 -> Bus Selector/1
  actuators/1 -> Bus Selector2/1

== system mainprueba3/LIBIS Plant/Aerodynamics/Cm ==
  prelook-ups : Inport
  plantData : Inport  Port=2
  actuators1 : Inport  Port=3
  Add1 : Sum  Inputs=+++++++
  Bus Selector : BusSelector  OutputSignals=alpha,alpha_dot,Omega_body.q
  Bus Selector1 : BusSelector  OutputSignals=alpha,alt,xcg,deltae,deltar,deltafr,deltafl
  Bus Selector3 : BusSelector  OutputSignals=deltae,deltafr,deltafl
  Cm0 : Interpolation_n-D  NumberOfTableDimensions=7  Table=LD.Stability.Cm0  RequireIndexFractionAsBus=on  InternalRulePriority=Speed
      settings: InputPortMap=u0,u1,u2,u3,u4,u5,u6
  Cmalpha : Interpolation_n-D  NumberOfTableDimensions=7  Table=LD.Stability.Cmalpha  RequireIndexFractionAsBus=on  InternalRulePriority=Speed
      settings: InputPortMap=u0,u1,u2,u3,u4,u5,u6
  Cmalpha_dot : Interpolation_n-D  NumberOfTableDimensions=7  Table=LD.Stability.Cmalpha_dot  RequireIndexFractionAsBus=on  InternalRulePriority=Speed
      settings: InputPortMap=u0,u1,u2,u3,u4,u5,u6
  Cmdeltae : Interpolation_n-D  NumberOfTableDimensions=7  Table=LD.Stability.Cmdeltae  RequireIndexFractionAsBus=on  InternalRulePriority=Speed
      settings: InputPortMap=u0,u1,u2,u3,u4,u5,u6
  Cmdeltafl : Interpolation_n-D  NumberOfTableDimensions=7  Table=LD.Stability.Cmdeltafl  RequireIndexFractionAsBus=on  InternalRulePriority=Speed
      settings: InputPortMap=u0,u1,u2,u3,u4,u5,u6
  Cmdeltafr : Interpolation_n-D  NumberOfTableDimensions=7  Table=LD.Stability.Cmdeltafr  RequireIndexFractionAsBus=on  InternalRulePriority=Speed
      settings: InputPortMap=u0,u1,u2,u3,u4,u5,u6
  Cmq : Interpolation_n-D  NumberOfTableDimensions=7  Table=LD.Stability.Cmq  RequireIndexFractionAsBus=on  InternalRulePriority=Speed
      settings: InputPortMap=u0,u1,u2,u3,u4,u5,u6
  Product{,1..5} (6 alike) : Product
  Cm : Outport
  wires:
  prelook-ups/1 -> Bus Selector1/1
  Cm0/1 -> Add1/1
  Add1/1 -> Cm/1
  Cmalpha/1 -> Product/1
  Cmalpha_dot/1 -> Product1/1
  Cmq/1 -> Product2/1
  Cmdeltae/1 -> Product3/1
  Product/1 -> Add1/2
  Product1/1 -> Add1/3
  Product2/1 -> Add1/4
  Product3/1 -> Add1/5
  Bus Selector/1 -> Product/2  "<alpha>"
  Bus Selector/2 -> Product1/2  "<alpha_dot>"
  Bus Selector/3 -> Product2/2  "<q>"
  plantData/1 -> Bus Selector/1
  actuators1/1 -> Bus Selector3/1
  Bus Selector3/3 -> Product5/2  "<deltafl>"
  Cmdeltafl/1 -> Product5/1
  Product5/1 -> Add1/7
  Product4/1 -> Add1/6
  Cmdeltafr/1 -> Product4/1
  Bus Selector3/2 -> Product4/2  "<deltafr>"
  Bus Selector3/1 -> Product3/2  "<deltae>"
  Bus Selector1/7 -> Cm0/7, Cmalpha/7, Cmalpha_dot/7, Cmdeltafl/7, Cmdeltafr/7, Cmdeltae/7, Cmq/7  "<deltafl>"
  Bus Selector1/6 -> Cm0/6, Cmalpha/6, Cmalpha_dot/6, Cmdeltafl/6, Cmdeltafr/6, Cmdeltae/6, Cmq/6  "<deltafr>"
  Bus Selector1/5 -> Cm0/5, Cmalpha/5, Cmalpha_dot/5, Cmdeltafl/5, Cmdeltafr/5, Cmdeltae/5, Cmq/5  "<deltar>"
  Bus Selector1/4 -> Cm0/4, Cmalpha/4, Cmalpha_dot/4, Cmdeltafl/4, Cmdeltafr/4, Cmdeltae/4, Cmq/4  "<deltae>"
  Bus Selector1/2 -> Cm0/2, Cmalpha/2, Cmalpha_dot/2, Cmq/2, Cmdeltafl/2, Cmdeltafr/2, Cmdeltae/2  "<alt>"
  Bus Selector1/3 -> Cm0/3, Cmalpha/3, Cmalpha_dot/3, Cmdeltafl/3, Cmdeltafr/3, Cmdeltae/3, Cmq/3  "<xcg>"
  Bus Selector1/1 -> Cm0/1, Cmalpha/1, Cmalpha_dot/1, Cmq/1, Cmdeltafl/1, Cmdeltafr/1, Cmdeltae/1  "<alpha>"

== system mainprueba3/LIBIS Plant/Aerodynamics/Cn ==
  prelook-ups : Inport
  plantData : Inport  Port=2
  actuators : Inport  Port=3
  Add : Sum  Inputs=++++++
  Bus Selector : BusSelector  OutputSignals=beta,Omega_body.p,Omega_body.r
  Bus Selector1 : BusSelector  OutputSignals=alpha,alt,xcg,deltae,deltar,deltafr,deltafl
  Bus Selector2 : BusSelector  OutputSignals=deltar,deltafr,deltafl
  Cnbeta : Interpolation_n-D  NumberOfTableDimensions=7  Table=LD.Stability.Cnbeta  RequireIndexFractionAsBus=on  InternalRulePriority=Speed
      settings: InputPortMap=u0,u1,u2,u3,u4,u5,u6
  "Cndeltafl " : Interpolation_n-D  NumberOfTableDimensions=7  Table=LD.Stability.Cndeltafl  RequireIndexFractionAsBus=on  InternalRulePriority=Speed
      settings: InputPortMap=u0,u1,u2,u3,u4,u5,u6
  "Cndeltafr " : Interpolation_n-D  NumberOfTableDimensions=7  Table=LD.Stability.Cndeltafr  RequireIndexFractionAsBus=on  InternalRulePriority=Speed
      settings: InputPortMap=u0,u1,u2,u3,u4,u5,u6
  Cndeltar : Interpolation_n-D  NumberOfTableDimensions=7  Table=LD.Stability.Cndeltar  RequireIndexFractionAsBus=on  InternalRulePriority=Speed
      settings: InputPortMap=u0,u1,u2,u3,u4,u5,u6
  Cnp : Interpolation_n-D  NumberOfTableDimensions=7  Table=LD.Stability.Cnp  RequireIndexFractionAsBus=on  InternalRulePriority=Speed
      settings: InputPortMap=u0,u1,u2,u3,u4,u5,u6
  Cnr : Interpolation_n-D  NumberOfTableDimensions=7  Table=LD.Stability.Cnr  RequireIndexFractionAsBus=on  InternalRulePriority=Speed
      settings: InputPortMap=u0,u1,u2,u3,u4,u5,u6
  Product{,1..5} (6 alike) : Product
  Cn : Outport
  wires:
  Bus Selector1/7 -> Cnp/7, Cnr/7, Cndeltar/7, "Cndeltafr "/7, "Cndeltafl "/7, Cnbeta/7  "<deltafl>"
  Bus Selector1/6 -> Cnp/6, Cnr/6, Cndeltar/6, "Cndeltafr "/6, "Cndeltafl "/6, Cnbeta/6  "<deltafr>"
  Bus Selector1/5 -> Cnp/5, Cnr/5, Cndeltar/5, "Cndeltafr "/5, "Cndeltafl "/5, Cnbeta/5  "<deltar>"
  prelook-ups/1 -> Bus Selector1/1
  Bus Selector1/4 -> Cnp/4, Cnr/4, Cndeltar/4, "Cndeltafr "/4, "Cndeltafl "/4, Cnbeta/4  "<deltae>"
  Bus Selector1/2 -> Cnp/2, Cnr/2, Cndeltar/2, "Cndeltafr "/2, "Cndeltafl "/2, Cnbeta/2  "<alt>"
  Bus Selector1/3 -> Cnp/3, Cnr/3, Cndeltar/3, "Cndeltafr "/3, "Cndeltafl "/3, Cnbeta/3  "<xcg>"
  Bus Selector1/1 -> Cnp/1, Cnr/1, Cndeltar/1, "Cndeltafr "/1, "Cndeltafl "/1, Cnbeta/1  "<alpha>"
  Add/1 -> Cn/1
  plantData/1 -> Bus Selector/1
  actuators/1 -> Bus Selector2/1
  Cnbeta/1 -> Product/1
  Product/1 -> Add/1
  Bus Selector/1 -> Product/2  "<beta>"
  Bus Selector2/1 -> Product3/2  "<deltar>"
  Cndeltar/1 -> Product3/1
  Product3/1 -> Add/4
  Product2/1 -> Add/3
  Product1/1 -> Add/2
  Cnp/1 -> Product1/1
  Cnr/1 -> Product2/1
  Bus Selector/3 -> Product2/2  "<r>"
  Bus Selector/2 -> Product1/2  "<p>"
  "Cndeltafl "/1 -> Product5/1
  Product5/1 -> Add/6
  Product4/1 -> Add/5
  "Cndeltafr "/1 -> Product4/1
  Bus Selector2/2 -> Product4/2  "<deltafr>"
  Bus Selector2/3 -> Product5/2  "<deltafl>"

== system mainprueba3/LIBIS Plant/Aerodynamics/DerivedConditions ==
  Speed of Sound : Inport
  Air Density : Inport  Port=2
  WindVelocity : Inport  Port=3  PortDimensions=3
  WindAngularRates : Inport  Port=4  PortDimensions=3
  Vb : Inport  Port=5  PortDimensions=3
  Dynamic Pressure : aerolibasang/Dynamic Pressure
  Mach Number : aerolibasang/Mach Number
  Sum2 : Sum  Inputs=|+-  SaturateOnIntegerOverflow=on  InputSameDT=on  OutDataTypeStr=Inherit: Same as first input
  Mach : Outport
  qbar : Outport  Port=2  InitialOutput=0
  "pqrWind " : Outport  Port=3
  wires:
  Speed of Sound/1 -> Mach Number/2  "speedSound"
  Mach Number/1 -> Mach/1  "Mach"
  Air Density/1 -> Dynamic Pressure/2
  Dynamic Pressure/1 -> qbar/1  "qbar"
  WindAngularRates/1 -> "pqrWind "/1
  Vb/1 -> Sum2/1  "V_body"
  Sum2/1 -> Dynamic Pressure/1, Mach Number/1  "V_ground"
  WindVelocity/1 -> Sum2/2  "V_wind"

== system mainprueba3/LIBIS Plant/Propulsion/8S 25C Battery ==
  note: ZIPPY Compact 5800mAh 8S 25C Lipo Pack
      |
      | Spec.
      | Capacity: 5800mAh
      | Voltage: 8S1P / 8 Cell / 29.6V
      | Discharge: 25C Constant / 35C Burst
      | Weight: 1025g (including wire, plug & case)
      | Dimensions: 167x46x64mm
      | Balance Plug: JST-XH
      | Discharge Plug: 5.5mm Bullet
  note: ZIPPY Compact 5800mAh 8S 25C Lipo Pack
      |
      | SKU
      | ZC.5800.8S.25
      | Weight(g):
      | 1020.00
      | Length:
      | 161.00
      | Width
      | 46.00
      | Height
      | 73.00
      | Capacity (mAh):
      | 5800.00
      | Discharge(c):
      | 25.00
      | Length-A(mm)
      | 167.00
      | Height-B(mm)
      | 46.00
      | Width-C(mm):
      | 64.00
      | Unit Weight (g):
      | 1020
      | Max Charge Rate(C)
      | 5.00
      | Watt Hour
      | 171.00
  note: Batería escogida: 8S 29.6V
  Battery_Capacity : Constant  Value=5.8
  Battery_Voltage : Constant  Value=29.6
  Max_discharge_rate : Constant  Value=145
  profundidad_descarga : Constant  Value=0.95
  rendimiento_bateria : Constant  Value=0.98
  V_battery : Outport  Unit=V
  C_battery : Outport  Port=2  Unit=A*h
  max_discharge_rate : Outport  Port=3  Unit=A*h
  deep_discharge_battery : Outport  Port=4  Unit=1
  eta_battery : Outport  Port=5  Unit=1
  wires:
  Battery_Voltage/1 -> V_battery/1
  Battery_Capacity/1 -> C_battery/1
  profundidad_descarga/1 -> deep_discharge_battery/1
  rendimiento_bateria/1 -> eta_battery/1
  Max_discharge_rate/1 -> max_discharge_rate/1
